simulink model "SIMULINK_EX_V_slx"  (R2021a)
settings: Solver=VariableStepAuto  StartTime=0.0  StopTime=10.0  RelTol=1e-3
settings Model: Creator=GHOST  LastModifiedBy=GHOST

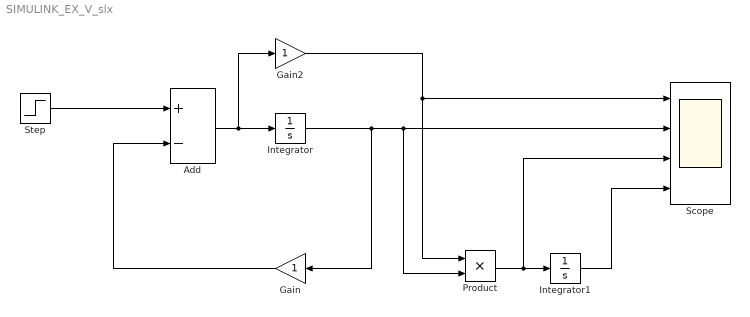
== system SIMULINK_EX_V_slx ==
  Add : Sum  Inputs=+-
  Gain : Gain
  Gain2 : Gain
  Integrator : Integrator
  Integrator1 : Integrator
  Product : Product
  Scope : Scope  NumInputPorts=4
  Step : Step  Before=1  SampleTime=0
  wires:
  Step/1 -> Add/1
  Add/1 -> Gain2/1, Integrator/1
  Integrator/1 -> Gain/1, Product/2, Scope/2
  Gain2/1 -> Product/1, Scope/1
  Integrator1/1 -> Scope/4
  Product/1 -> Integrator1/1, Scope/3
  Gain/1 -> Add/2
